simulink model "ohc_calc_tau"  (R2020b)
settings: Solver=FixedStepDiscrete  StartTime=0.0  StopTime=stopTime  RelTol=1e-3
InitFcn:
  | initCallback
StopFcn:
  | stopCallback
values from neighbouring files (symbols this model uses):
  bmTaumax = taumax/bwfactor    (= 0.0030112115233)    [modelparameters.m]
  bmTaumin = bmTaumax*ratio_taubm    (= 0.00150918077323)    [modelparameters.m]
  centerfreq = 165.4*(10^((bmplace+1.2)/(35/2.1))-1.0)    [modelparameters.m]
  cf = 1000    [modelparameters.m]
  cohc = 1    [modelparameters.m]
  tauwb_i = TauWBMax+(bmTaubm-bmTaumax)*(TauWBMax-TauWBMin)/(bmTaumax-bmTaumin)    (= 0.00136983367319)    [modelparameters.m]
  TauWBMax = taumin+0.2*(taumax-taumin)    (= 0.00136983367319)    [modelparameters.m]
  TauWBMin = TauWBMax/taumax*taumin    (= 0.000770314083071)    [modelparameters.m]
  tdres = 1/Fs    (= 2.08333333333e-05)    [modelparameters.m]
  TWOPI = 6.28318530717959    (= 6.28318530718)    [modelparameters.m]
undefined symbols (not defined in the file or in its folder): mp, wbgain_i
libraries: hdlsllib x2, simulink x1
settings Model: Creator=Ross  LastModifiedBy=wickh
settings DataIOCC: ReturnWorkspaceOutputs=off
settings OptimizationCC: BlockReduction=off  ConditionallyExecuteInputs=off  DefaultParameterBehavior=Inlined
settings DebuggingCC: ReadBeforeWriteMsg=DisableAll  WriteAfterWriteMsg=DisableAll  WriteAfterReadMsg=DisableAll  AlgebraicLoopMsg=error  MultiTaskDSMMsg=none  SingleTaskRateTransMsg=error  PregeneratedLibrarySubsystemCodeDiagnostic=none  ArithmeticOperatorsInVariantConditions=warning
settings HardwareCC: ProdBitPerPointer=32  ProdBitPerSizeT=32  ProdBitPerPtrDiffT=32  ProdLargestAtomicFloat=None  ProdIntDivRoundTo=Undefined  ProdEndianess=Unspecified  ProdWordSize=32  ProdHWDeviceType=ASIC/FPGA->ASIC/FPGA  TargetBitPerPointer=64  TargetBitPerSizeT=64  TargetBitPerPtrDiffT=64  TargetLongLongMode=on  TargetIntDivRoundTo=Zero  TargetEndianess=LittleEndian  TargetWordSize=64  TargetHWDeviceType=Custom Processor->MATLAB Host Computer  ProdEqTarget=off
settings ModelReferenceCC: UpdateModelReferenceTargets=IfOutOfDate
settings SFSimCC: SFSimEcho=off  SimUseLocalCustomCode=off  CustomCodeUndefinedFunction=UseInterfaceOnly
settings RTWCC: RTWUseLocalCustomCode=off

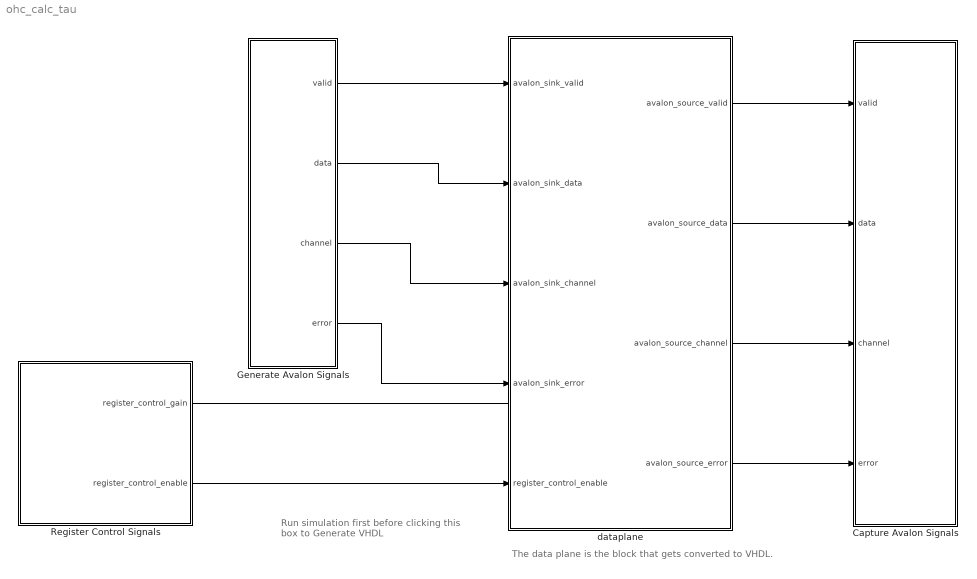
== system ohc_calc_tau ==
  note: The data plane is the block that gets converted to VHDL.
  note: Run simulation first
      | before clicking this box to
      | Generate VHDL
  Capture Avalon Signals : Subsystem
  Generate Avalon Signals : Subsystem
  Register Control Signals : Subsystem
  dataplane : Subsystem  TreatAsAtomicUnit=on
  wires:
  Generate Avalon Signals/2(data) -> dataplane/2(avalon_sink_data)
  Generate Avalon Signals/1(valid) -> dataplane/1(avalon_sink_valid)
  Generate Avalon Signals/3(channel) -> dataplane/3(avalon_sink_channel)
  Generate Avalon Signals/4(error) -> dataplane/4(avalon_sink_error)
  dataplane/2(avalon_source_data) -> Capture Avalon Signals/2(data)
  dataplane/1(avalon_source_valid) -> Capture Avalon Signals/1(valid)
  dataplane/3(avalon_source_channel) -> Capture Avalon Signals/3(channel)
  dataplane/4(avalon_source_error) -> Capture Avalon Signals/4(error)
  Register Control Signals/1(register_control_gain) -> ?
  Register Control Signals/2(register_control_enable) -> dataplane/5(register_control_enable)

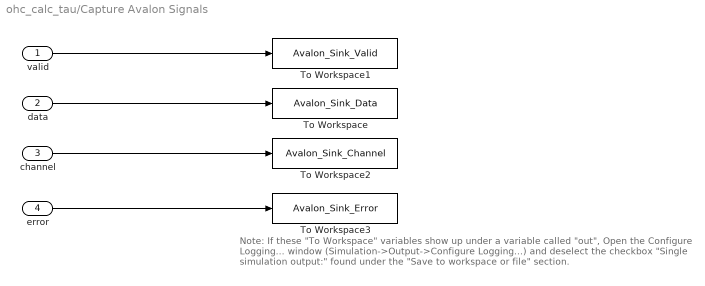
== system ohc_calc_tau/Capture Avalon Signals ==
  note: Note:  If these "To Workspace" variables show up under a variable called "out",
      | Open the Configure Logging... window (Simulation->Output->Configure Logging...)
      | and deselect the checkbox "Single simulation output:" found under the "Save to workspace or file" section.
  valid : Inport
  data : Inport  Port=2
  channel : Inport  Port=3
  error : Inport  Port=4
  To Workspace : ToWorkspace  VariableName=Avalon_Sink_Data  SaveFormat=Timeseries  SampleTime=-1
  To Workspace1 : ToWorkspace  VariableName=Avalon_Sink_Valid  SaveFormat=Timeseries  SampleTime=-1
  To Workspace2 : ToWorkspace  VariableName=Avalon_Sink_Channel  SaveFormat=Timeseries  SampleTime=-1
  To Workspace3 : ToWorkspace  VariableName=Avalon_Sink_Error  SaveFormat=Timeseries  SampleTime=-1
  wires:
  data/1 -> To Workspace/1
  valid/1 -> To Workspace1/1
  error/1 -> To Workspace3/1
  channel/1 -> To Workspace2/1

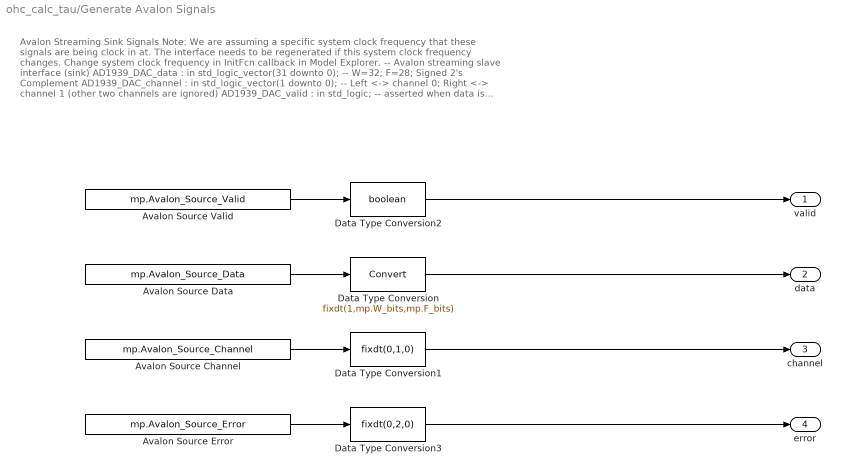
== system ohc_calc_tau/Generate Avalon Signals ==
  note: Avalon Streaming Sink Signals
      | Note: We are assuming a specific system clock frequency that these signals are being clock in at.
      | The interface needs to be regenerated if this system clock frequency changes. Change system clock frequency in InitFcn callback in Model Explorer.
      |
      | -- Avalon streaming slave interface (sink)
      | AD1939_DAC_data : in std_logic_vector(31 downto 0); -- W=32; F=28; Signed 2's Complement
      | AD1939_DAC_channel : in std_logic_vector(1 downto 0); -- Left <-> channel 0; Right <-> channel 1 (other two channels are ignored)
      | AD1939_DAC_valid : in std_logic; -- asserted when data is valid
      | AD1939_DAC_error : in std_logic_vector(1 downto 0) -- error channel is ignored, assumed to be error free at this point
      |
      | For more information on the data-channel-valid protocol, s ee chapter 5 in Intel's Avalon Interfaced Specification (p. 40) at https://www.intel.com/content/dam/www/programmable/us/en/pdfs/literature/manual/mnl_avalon_spec.pdf
  Avalon Source Channel : FromWorkspace  VariableName=mp.Avalon_Source_Channel  OutDataTypeStr=double  SampleTime=mp.Ts_sim
  "Avalon Source Data " : FromWorkspace  VariableName=mp.Avalon_Source_Data  OutDataTypeStr=double  SampleTime=mp.Ts_sim
  Avalon Source Error : FromWorkspace  VariableName=mp.Avalon_Source_Error  OutDataTypeStr=double  SampleTime=mp.Ts_sim
  Avalon Source Valid : FromWorkspace  VariableName=mp.Avalon_Source_Valid  OutDataTypeStr=double  SampleTime=mp.Ts_sim
  Data Type Conversion : DataTypeConversion  OutDataTypeStr=fixdt(1,mp.W_bits,mp.F_bits)
  Data Type Conversion1 : DataTypeConversion  OutDataTypeStr=fixdt(0,1,0)
  Data Type Conversion2 : DataTypeConversion  OutDataTypeStr=boolean
  Data Type Conversion3 : DataTypeConversion  OutDataTypeStr=fixdt(0,2,0)
  valid : Outport  VectorParamsAs1DForOutWhenUnconnected=off
  data : Outport  Port=2  VectorParamsAs1DForOutWhenUnconnected=off
  channel : Outport  Port=3  VectorParamsAs1DForOutWhenUnconnected=off
  error : Outport  Port=4  VectorParamsAs1DForOutWhenUnconnected=off
  wires:
  Data Type Conversion1/1 -> channel/1
  Data Type Conversion2/1 -> valid/1
  Avalon Source Error/1 -> Data Type Conversion3/1
  Data Type Conversion/1 -> data/1
  Avalon Source Valid/1 -> Data Type Conversion2/1
  Data Type Conversion3/1 -> error/1
  Avalon Source Channel/1 -> Data Type Conversion1/1
  "Avalon Source Data "/1 -> Data Type Conversion/1

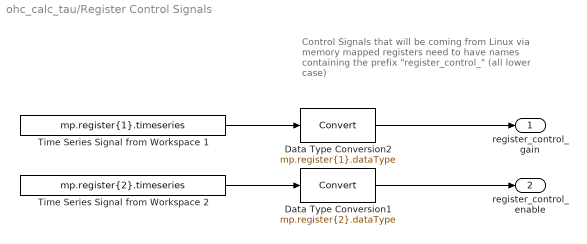
== system ohc_calc_tau/Register Control Signals ==
  note: Control Signals that will be coming from Linux via
      | memory mapped registers need to have names
      | containing the prefix "register_control_"
      | (all lower case)
  Data Type Conversion1 : DataTypeConversion  OutDataTypeStr=mp.register{2}.dataType
  Data Type Conversion2 : DataTypeConversion  OutDataTypeStr=mp.register{1}.dataType
  Time Series Signal from Workspace 1 : FromWorkspace  VariableName=mp.register{1}.timeseries  OutDataTypeStr=double  SampleTime=mp.Ts_sim
  Time Series Signal from Workspace 2 : FromWorkspace  VariableName=mp.register{2}.timeseries  OutDataTypeStr=double  SampleTime=mp.Ts_sim
  register_control_gain : Outport  VectorParamsAs1DForOutWhenUnconnected=off
  register_control_enable : Outport  Port=2  VectorParamsAs1DForOutWhenUnconnected=off
  wires:
  Time Series Signal from Workspace 1/1 -> Data Type Conversion2/1
  Data Type Conversion2/1 -> register_control_gain/1
  Data Type Conversion1/1 -> register_control_enable/1
  Time Series Signal from Workspace 2/1 -> Data Type Conversion1/1

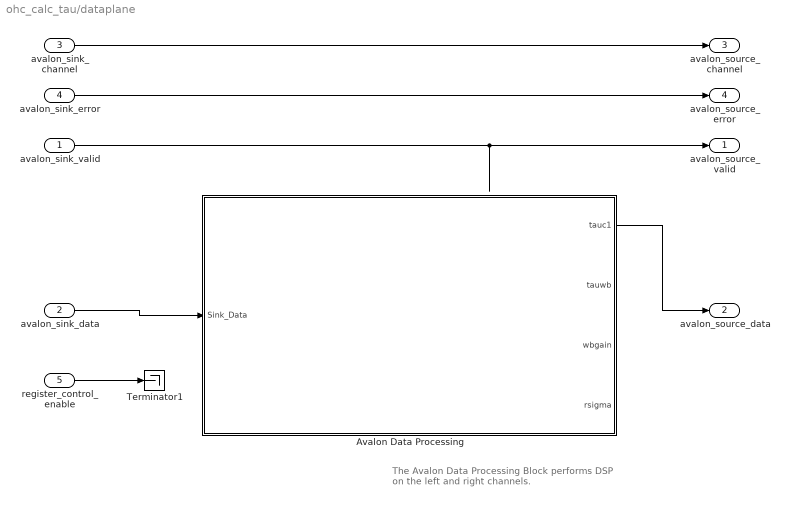
== system ohc_calc_tau/dataplane ==
  note: The Avalon Data Processing Block
      | performs DSP on the left and right channels.
  avalon_sink_valid : Inport
  avalon_sink_data : Inport  Port=2
  avalon_sink_channel : Inport  Port=3
  avalon_sink_error : Inport  Port=4
  register_control_enable : Inport  Port=5
  Avalon Data Processing : Subsystem  TreatAsAtomicUnit=on
  Terminator1 : Terminator
  avalon_source_valid : Outport  VectorParamsAs1DForOutWhenUnconnected=off
  avalon_source_data : Outport  Port=2  VectorParamsAs1DForOutWhenUnconnected=off
  avalon_source_channel : Outport  Port=3  VectorParamsAs1DForOutWhenUnconnected=off
  avalon_source_error : Outport  Port=4  VectorParamsAs1DForOutWhenUnconnected=off
  wires:
  avalon_sink_error/1 -> avalon_source_error/1
  avalon_sink_valid/1 -> avalon_source_valid/1
  avalon_sink_data/1 -> Avalon Data Processing/1(Sink_Data)
  Avalon Data Processing/1(tauc1) -> avalon_source_data/1
  avalon_sink_channel/1 -> avalon_source_channel/1
  register_control_enable/1 -> Terminator1/1

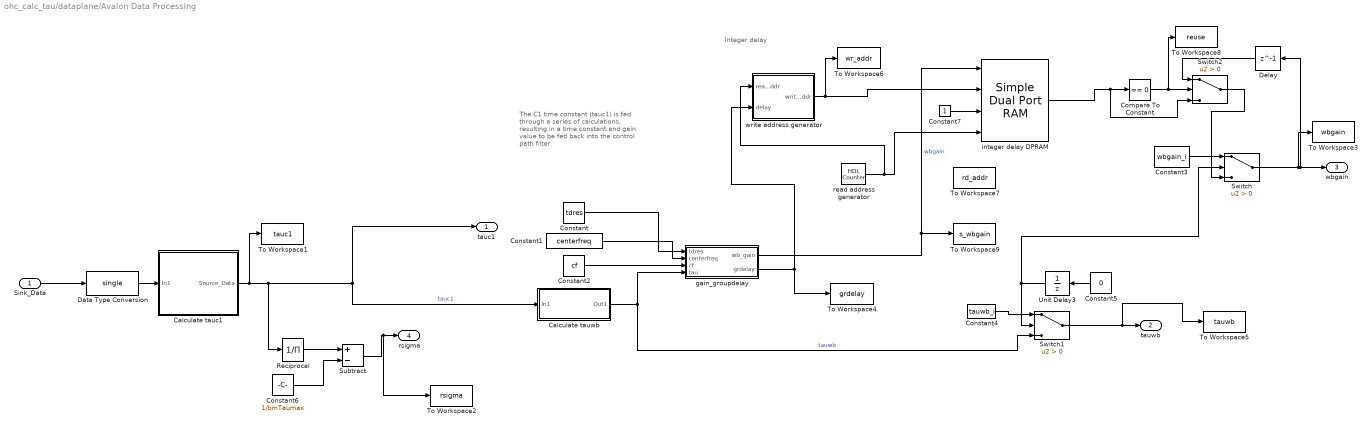
== system ohc_calc_tau/dataplane/Avalon Data Processing ==
  note: The C1 time constant (tauc1) is fed through a series of calculations, resulting in a time constant and gain value to be fed back into the control path filter
  note: Integer delay
  Sink_Data : Inport
  Calculate tauc1 : Subsystem
  Calculate tauwb : Subsystem
  Compare To Constant : simulink/Logic and Bit Operations/Compare To Constant  relop===  const=0  OutDataTypeStr=boolean
  Constant : Constant  Value=tdres  OutDataTypeStr=single  SampleTime=-1
  Constant1 : Constant  Value=centerfreq  OutDataTypeStr=single  SampleTime=-1
  Constant2 : Constant  Value=cf  OutDataTypeStr=single  SampleTime=-1
  Constant3 : Constant  Value=wbgain_i  OutDataTypeStr=single  SampleTime=-1
  Constant4 : Constant  Value=tauwb_i  OutDataTypeStr=single  SampleTime=-1
  Constant5 : Constant  Value=0  OutDataTypeStr=single  SampleTime=-1
  Constant6 : Constant  Value=1/bmTaumax  OutDataTypeStr=single  SampleTime=-1
  Constant7 : Constant  OutDataTypeStr=Inherit: Inherit via back propagation  SampleTime=-1
  Data Type Conversion : DataTypeConversion  OutDataTypeStr=single
  Delay : Delay  DelayLength=1
  Reciprocal : Product  Inputs=/  RndMeth=Zero  SaturateOnIntegerOverflow=on
  Subtract : Sum  Inputs=+-
  Switch : Switch  Criteria=u2 > Threshold
  Switch1 : Switch  Criteria=u2 > Threshold
  Switch2 : Switch  Criteria=u2 > Threshold
  To Workspace1 : ToWorkspace  VariableName=tauc1  SampleTime=-1
      settings: Save2DSignal=2-D array (concatenate along first dimension)
  To Workspace2 : ToWorkspace  VariableName=rsigma  SampleTime=-1
      settings: Save2DSignal=2-D array (concatenate along first dimension)
  To Workspace3 : ToWorkspace  VariableName=wbgain  SampleTime=-1
      settings: Save2DSignal=2-D array (concatenate along first dimension)
  To Workspace4 : ToWorkspace  VariableName=grdelay  SampleTime=-1
      settings: Save2DSignal=2-D array (concatenate along first dimension)
  To Workspace5 : ToWorkspace  VariableName=tauwb  SampleTime=-1
      settings: Save2DSignal=2-D array (concatenate along first dimension)
  To Workspace6 : ToWorkspace  VariableName=wr_addr  SampleTime=-1
      settings: Save2DSignal=2-D array (concatenate along first dimension)
  To Workspace7 : ToWorkspace  VariableName=rd_addr  SampleTime=-1
      settings: Save2DSignal=2-D array (concatenate along first dimension)
  To Workspace8 : ToWorkspace  VariableName=reuse  SampleTime=-1
      settings: Save2DSignal=2-D array (concatenate along first dimension)
  To Workspace9 : ToWorkspace  VariableName=s_wbgain  SampleTime=-1
      settings: Save2DSignal=2-D array (concatenate along first dimension)
  Unit Delay3 : UnitDelay  InitialCondition=1  SampleTime=-1  HasFrameUpgradeWarning=on
  gain_groupdelay : Subsystem
  integer delay DPRAM : hdlsllib/HDL RAMs/Simple Dual Port RAM  ram_size=mp.integerDelayAddrSize
      settings: SourceProductBaseCode=SL
  read address generator : hdlsllib/Sources/HDL Counter  CountType=Count limited  CountInit=0  CountStep=1  CountMax=mp.integerDelayBufferSize - 1  CountFromType=Initial value  CountFrom=0  CountResetPort=off  CountLoadPort=off  CountEnbPort=off  CountDirPort=off  CountDataType=Unsigned  CountWordLen=mp.integerDelayAddrSize  CountFracLen=0  CountSampTime=-1
  write address generator : Subsystem
  tauc1 : Outport  InitialOutput=0  VectorParamsAs1DForOutWhenUnconnected=off
  tauwb : Outport  Port=2  VectorParamsAs1DForOutWhenUnconnected=off
  wbgain : Outport  Port=3  VectorParamsAs1DForOutWhenUnconnected=off
  rsigma : Outport  Port=4  VectorParamsAs1DForOutWhenUnconnected=off
  wires:
  Sink_Data/1 -> Data Type Conversion/1
  Data Type Conversion/1 -> Calculate tauc1/1(In1)
  Calculate tauc1/1(Source_Data) -> Reciprocal/1, Calculate tauwb/1(In1), tauc1/1, To Workspace1/1  "tauc1"
  Constant5/1 -> Unit Delay3/1
  Switch/1 -> Delay/1, wbgain/1, To Workspace3/1
  Unit Delay3/1 -> Switch/2, Switch1/2
  Constant3/1 -> Switch/1
  Constant/1 -> gain_groupdelay/1(tdres)
  Switch1/1 -> To Workspace5/1, tauwb/1
  Calculate tauwb/1(Out1) -> gain_groupdelay/4(tau), Switch1/3  "tauwb"
  Constant4/1 -> Switch1/1
  Constant2/1 -> gain_groupdelay/3(cf)
  Constant1/1 -> gain_groupdelay/2(centerfreq)
  integer delay DPRAM/1 -> Switch2/3, Compare To Constant/1
  Reciprocal/1 -> Subtract/1
  Constant6/1 -> Subtract/2
  Subtract/1 -> To Workspace2/1, rsigma/1
  gain_groupdelay/2(grdelay) -> To Workspace4/1, write address generator/2(delay)
  Constant7/1 -> integer delay DPRAM/3
  gain_groupdelay/1(wb_gain) -> To Workspace9/1, integer delay DPRAM/1  "wbgain"
  Compare To Constant/1 -> To Workspace8/1, Switch2/2
  Switch2/1 -> Switch/3
  Delay/1 -> Switch2/1
  read address generator/1 -> write address generator/1(read_addr), integer delay DPRAM/4
  write address generator/1(write_addr) -> integer delay DPRAM/2, To Workspace6/1

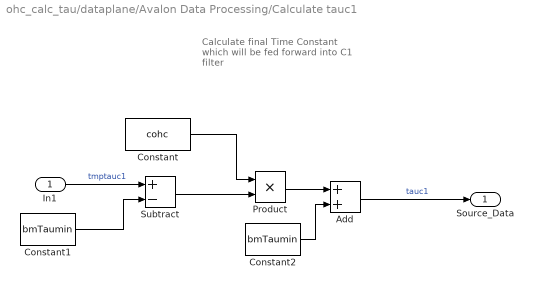
== system ohc_calc_tau/dataplane/Avalon Data Processing/Calculate tauc1 ==
  note: Calculate final Time Constant which will be fed forward into C1 filter
  In1 : Inport
  Add : Sum
  Constant : Constant  Value=cohc  OutDataTypeStr=single  SampleTime=-1
  Constant1 : Constant  Value=bmTaumin  OutDataTypeStr=single  SampleTime=-1
  Constant2 : Constant  Value=bmTaumin  OutDataTypeStr=single  SampleTime=-1
  Product : Product
  Subtract : Sum  Inputs=+-
  Source_Data : Outport  VectorParamsAs1DForOutWhenUnconnected=off
  wires:
  In1/1 -> Subtract/1  "tmptauc1"
  Constant/1 -> Product/1
  Constant1/1 -> Subtract/2
  Product/1 -> Add/1
  Add/1 -> Source_Data/1  "tauc1"
  Subtract/1 -> Product/2
  Constant2/1 -> Add/2

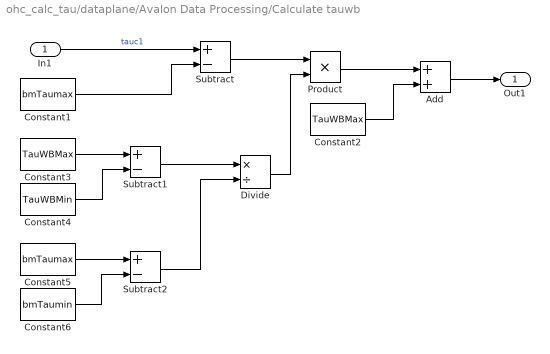
== system ohc_calc_tau/dataplane/Avalon Data Processing/Calculate tauwb ==
  In1 : Inport
  Add : Sum
  Constant1 : Constant  Value=bmTaumax  OutDataTypeStr=single  SampleTime=-1
  Constant2 : Constant  Value=TauWBMax  OutDataTypeStr=single  SampleTime=-1
  Constant3 : Constant  Value=TauWBMax  OutDataTypeStr=single  SampleTime=-1
  Constant4 : Constant  Value=TauWBMin  OutDataTypeStr=single  SampleTime=-1
  Constant5 : Constant  Value=bmTaumax  OutDataTypeStr=single  SampleTime=-1
  Constant6 : Constant  Value=bmTaumin  OutDataTypeStr=single  SampleTime=-1
  Divide : Product  Inputs=*/  RndMeth=Zero  SaturateOnIntegerOverflow=on
  Product : Product
  Subtract : Sum  Inputs=+-
  Subtract1 : Sum  Inputs=+-
  Subtract2 : Sum  Inputs=+-
  Out1 : Outport  OutDataTypeStr=single  VectorParamsAs1DForOutWhenUnconnected=off
  wires:
  In1/1 -> Subtract/1  "tauc1"
  Constant1/1 -> Subtract/2
  Product/1 -> Add/1
  Subtract/1 -> Product/1
  Constant3/1 -> Subtract1/1
  Constant4/1 -> Subtract1/2
  Constant6/1 -> Subtract2/2
  Constant5/1 -> Subtract2/1
  Subtract2/1 -> Divide/2
  Subtract1/1 -> Divide/1
  Divide/1 -> Product/2
  Constant2/1 -> Add/2
  Add/1 -> Out1/1

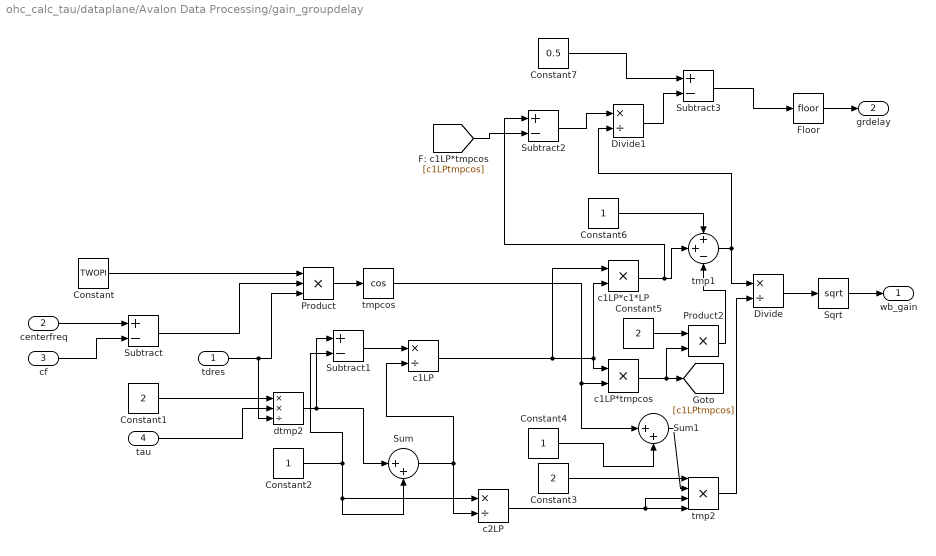
== system ohc_calc_tau/dataplane/Avalon Data Processing/gain_groupdelay ==
  tdres : Inport
  centerfreq : Inport  Port=2
  cf : Inport  Port=3
  tau : Inport  Port=4
  Constant : Constant  Value=TWOPI  OutDataTypeStr=single  SampleTime=-1
  Constant1 : Constant  Value=2  OutDataTypeStr=single  SampleTime=-1
  Constant2 : Constant  OutDataTypeStr=single  SampleTime=-1
  Constant3 : Constant  Value=2  OutDataTypeStr=single  SampleTime=-1
  Constant4 : Constant  OutDataTypeStr=single  SampleTime=-1
  Constant5 : Constant  Value=2  OutDataTypeStr=single  SampleTime=-1
  Constant6 : Constant  OutDataTypeStr=single  SampleTime=-1
  Constant7 : Constant  Value=0.5  OutDataTypeStr=single  SampleTime=-1
  Divide : Product  Inputs=*/  RndMeth=Zero  SaturateOnIntegerOverflow=on
  Divide1 : Product  Inputs=*/  RndMeth=Zero  SaturateOnIntegerOverflow=on
  Floor : Rounding
  Product : Product  Inputs=3
  Product2 : Product
  Sqrt : Sqrt  SaturateOnIntegerOverflow=on
  Subtract{,1..3} (4 alike) : Sum  Inputs=+-
  Sum : Sum  Inputs=|++
  Sum1 : Sum  Inputs=|++
  c1LP : Product  Inputs=*/
  c1LP*c1*LP : Product
  c1LP*tmpcos : Product
  c2LP : Product  Inputs=*/  RndMeth=Zero  SaturateOnIntegerOverflow=on
  dtmp2 : Product  Inputs=**/
  tmp1 : Sum  Inputs=++-
  tmp2 : Product  Inputs=4
  tmpcos : Trigonometry  Operator=cos
  wb_gain : Outport
  grdelay : Outport  Port=2
  wires:
  centerfreq/1 -> Subtract/1
  cf/1 -> Subtract/2
  Constant/1 -> Product/1
  Subtract/1 -> Product/2
  tdres/1 -> Product/3, dtmp2/3
  Product/1 -> tmpcos/1
  tau/1 -> dtmp2/2
  Constant1/1 -> dtmp2/1
  dtmp2/1 -> Sum/1, Subtract1/1
  Sum/1 -> c2LP/2, c1LP/2
  Constant2/1 -> c2LP/1, Sum/2, Subtract1/2
  Subtract1/1 -> c1LP/1
  Constant3/1 -> tmp2/1
  c2LP/1 -> tmp2/4, tmp2/3
  Constant4/1 -> Sum1/2
  tmpcos/1 -> Sum1/1, c1LP*tmpcos/2
  Sum1/1 -> tmp2/2
  c1LP/1 -> c1LP*c1*LP/2, c1LP*tmpcos/1, c1LP*c1*LP/1
  c1LP*tmpcos/1 -> [c1LPtmpcos], Product2/2
  c1LP*c1*LP/1 -> Subtract2/1, tmp1/2
  Constant6/1 -> tmp1/1
  tmp2/1 -> Divide/2
  Divide/1 -> Sqrt/1
  Sqrt/1 -> wb_gain/1
  Constant5/1 -> Product2/1
  Product2/1 -> tmp1/3
  [c1LPtmpcos] -> Subtract2/2
  Constant7/1 -> Subtract3/1
  Floor/1 -> grdelay/1
  tmp1/1 -> Divide1/2, Divide/1
  Subtract2/1 -> Divide1/1
  Divide1/1 -> Subtract3/2
  Subtract3/1 -> Floor/1

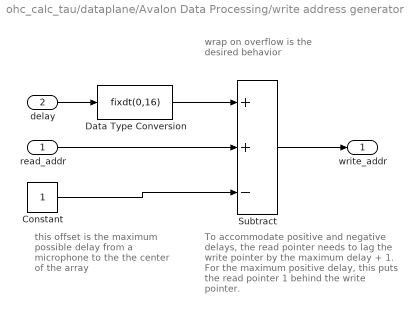
== system ohc_calc_tau/dataplane/Avalon Data Processing/write address generator ==
  note: To accommodate positive and negative delays, the read pointer needs to lag the write pointer by the maximum delay + 1. For the maximum positive delay, this puts the read pointer 1 behind the write pointer.
  note: this offset is the maximum possible delay from a microphone to the the center of the array
  note: wrap on overflow is the desired behavior
  read_addr : Inport
  delay : Inport  Port=2
  Constant : Constant  SampleTime=-1
  Data Type Conversion : DataTypeConversion  OutMin=0  OutMax=1024  OutDataTypeStr=fixdt(0,16)  RndMeth=Nearest
  Subtract : Sum  Inputs=++-  OutDataTypeStr=Inherit: Inherit via back propagation
  write_addr : Outport  VectorParamsAs1DForOutWhenUnconnected=off
  wires:
  delay/1 -> Data Type Conversion/1
  read_addr/1 -> Subtract/2
  Subtract/1 -> write_addr/1
  Data Type Conversion/1 -> Subtract/1
  Constant/1 -> Subtract/3
